simulink library "carnotUIBK_bus"  (R2023b)
settings: Solver=VariableStepAuto  StartTime=0.0  StopTime=10.0  RelTol=1e-3  EnableMultiTasking=on
values from neighbouring files (symbols this model uses):
  A = 7*10*2    (= 140)    [theta_ground_v1.m]    (also in xlswrite1.m = num2cell(data))
  amb_factor = 1    [DOOR.m]    (also in WALL.m; WINDOW.m = 0)
  area = obj.width * obj.height    [DOOR.m]    (also in RES.m = []; ROOM.m = 0; THERMALZONE.m = area + room(kk).area; WALL.m = area - obj.doors(jj).calc_area())
  B = A/(0.5 * P)    (= 8.23529411765)    [theta_ground_v1.m]
  boundary = BOUNDARY()    [BUILDING.m]    (also in WALL.m = '')
  building = obj    [BUILDING.m]    (also in create_building_automatic.m = building.save(); ini_building_automatic.m = building.add_variant_hvac(building.variant_hvac, hvac); load_building_automatic.m = building.save())
  C = zeros(1,length(d)+1)    [CONSTRUCTION.m]    (also in DOOR.m = [0 0 0]; WALL.m = [0 0 0]; WINDOW.m = [0 0 0])
  control = 2    [GAIN.m]    (also in GAINS.m)
  cp = str2num(value)    [CONSTRUCTION.m]
  height = 0    [DOOR.m]    (also in ROOM.m; THERMALZONE.m; WALL.m; WINDOW.m)
  p = [timevec_weather weather(:,12)]    [BOUNDARY.m]    (also in WEATHER.m = 0; init_carnotUIBK.m = cell2mat(carnotUIBKpaths(i,2)))
  rho = str2num(value)    [CONSTRUCTION.m]    (also in theta_ground_v1.m = 2000)
  type = 1    [CONSTRUCTION.m]    (also in GAINS.m = raw_moisture{ii,3}; STRUCTURE.m = 0)
  view_factor = 1    [DOOR.m]    (also in WINDOW.m = 0)
  wall = []    [ROOM.m]
  z = obj.Z    [WALL.m]    (also in theta_ground_v1.m = 0)
  zone = obj.zone(ind)    [THERMALZONE.m]
undefined symbols (not defined in the file or in its folder): const, Dd, get_building, mdot_air, mdot_CO2, mdot_H2O, mdot_VOC, pos, Qdot_C, Qdot_H, Qdot_I_electricity, Qdot_I_light, Qdot_I_person, Qdot_S, Qdot_T_ground, Qdot_T_internal, Qdot_T_neighbour, Qdot_T_opaque, Qdot_T_window, Qdot_V_infiltration, Qdot_V_mech, Qdot_V_window, Qdotc, Qdotr, r_frame, solar_ratio, solar_ratio1, solar_ratio2, Tc, Tr, Ts, Uvalue, wallsurface, window, window_height, window_heigth, window_width, windowsurface, x_CO2, x_H2O, x_VOC
libraries: $bdroot x134, carnot x87, simulink_extras x14, slpidlib x4, simulink x3
(part 4 of 12)

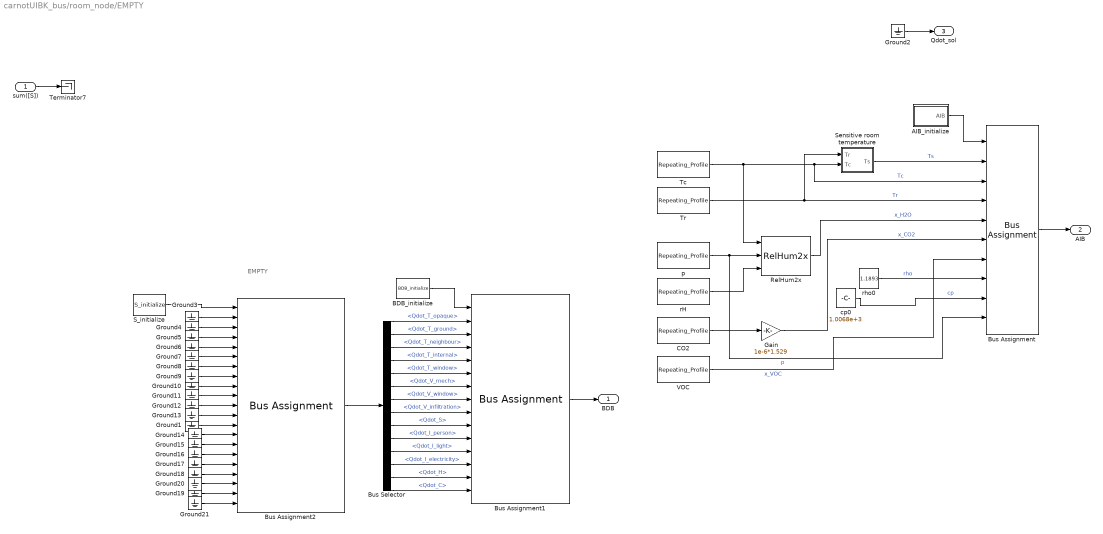
== system carnotUIBK_bus/room_node/EMPTY ==
  note: EMPTY
  sum([S]) : Inport
  AIB_initialize : Subsystem
  BDB_initialize : $bdroot/general/BDB_initialize  SystemSampleTime=-1  VariantActivationTime=update diagram  AllowFlexibleInterface=on  Latency=0  AutoFrameSizeCalculation=off
  Bus Assignment : BusAssignment  AssignedSignals=Ts,Tc,Tr,x_H2O,x_CO2,x_VOC,rho,cp,p
  Bus Assignment1 : BusAssignment  AssignedSignals=Qdot_T_opaque,Qdot_T_ground,Qdot_T_neighbour,Qdot_T_internal,Qdot_T_window,Qdot_V_mech,Qdot_V_window,Qdot_V_infiltration,Qdot_S,Qdot_I_person,Qdot_I_light,Qdot_I_electricity,Qdot_H,Qdot_C
  Bus Assignment2 : BusAssignment  AssignedSignals=Qdotc,Qdotr,Qdot_S,mdot_air,mdot_H2O,mdot_CO2,mdot_VOC,Qdot_T_opaque,Qdot_T_ground,Qdot_T_neighbour,Qdot_T_window,Qdot_T_internal,Qdot_V_mech,Qdot_V_window,Qdot_V_infiltration,Qdot_I_person,Qdot_I_light,Qdot_I_electricity,Qdot_H,Qdot_C
  Bus Selector : BusSelector  OutputSignals=Qdot_T_opaque,Qdot_T_ground,Qdot_T_neighbour,Qdot_T_internal,Qdot_T_window,Qdot_V_mech,Qdot_V_window,Qdot_V_infiltration,Qdot_S,Qdot_I_person,Qdot_I_light,Qdot_I_electricity,Qdot_H,Qdot_C
  CO2 : carnot/Load/General/Repeating_Profile  period=temperature_timevalues(end)  rep_seq_t=temperature_timevalues(1:end-1)  rep_seq_d=temperature_timeduration  rep_seq_y=temperature_CO2
      settings: SourceProductName=Carnot
  Gain : Gain  Gain=1e-6*1.529
  Ground{1..21} (21 alike) : Ground
  RelHum2x : carnot/Basic/Material_Properties/RelHum2x
      settings: SourceProductName=Carnot
  S_initialize : $bdroot/general/S_initialize  SystemSampleTime=-1  VariantActivationTime=update diagram  AllowFlexibleInterface=on  Latency=0  AutoFrameSizeCalculation=off
  Sensitive room temperature : Subsystem  mask(SENSITIVE TEMPERATURE){share_c=50}
      mask prompts: share_c "SHARE of convective part, [0,100%]:"
      mask help:
      | This block merges the convective and radiative zone node temperature to the SENSITIVE ZONE TEMPERATURE (weighted arithmetic average of both components).
      |
      | [T] = [Tc; Tr]:  temperature vector of node, °C
      | Ts:              sensitive zone temperature, °C
      mask init: same as carnotUIBK_bus/room_node/2-node/Sensitive room temperature
  Tc : carnot/Load/General/Repeating_Profile  period=temperature_timevalues(end)  rep_seq_t=temperature_timevalues(1:end-1)  rep_seq_d=temperature_timeduration  rep_seq_y=temperature_Tc
      settings: SourceProductName=Carnot
  Terminator7 : Terminator
  Tr : carnot/Load/General/Repeating_Profile  period=temperature_timevalues(end)  rep_seq_t=temperature_timevalues(1:end-1)  rep_seq_d=temperature_timeduration  rep_seq_y=temperature_Tr
      settings: SourceProductName=Carnot
  VOC : carnot/Load/General/Repeating_Profile  period=temperature_timevalues(end)  rep_seq_t=temperature_timevalues(1:end-1)  rep_seq_d=temperature_timeduration  rep_seq_y=temperature_VOC
      settings: SourceProductName=Carnot
  cp0 : Constant  Value=1.0068e+3
  p : carnot/Load/General/Repeating_Profile  period=temperature_timevalues(end)  rep_seq_t=temperature_timevalues(1:end-1)  rep_seq_d=temperature_timeduration  rep_seq_y=temperature_p
      settings: SourceProductName=Carnot
  rH : carnot/Load/General/Repeating_Profile  period=temperature_timevalues(end)  rep_seq_t=temperature_timevalues(1:end-1)  rep_seq_d=temperature_timeduration  rep_seq_y=temperature_rH
      settings: SourceProductName=Carnot
  rho0 : Constant  Value=1.1893
  BDB : Outport  VectorParamsAs1DForOutWhenUnconnected=off
  AIB : Outport  Port=2  VectorParamsAs1DForOutWhenUnconnected=off
  Qdot_sol : Outport  Port=3  VectorParamsAs1DForOutWhenUnconnected=off
  wires:
  Ground2/1 -> Qdot_sol/1
  cp0/1 -> Bus Assignment/9  "cp"
  rho0/1 -> Bus Assignment/8  "rho"
  p/1 -> Bus Assignment/10, RelHum2x/2  "p"
  VOC/1 -> Bus Assignment/7  "x_VOC"
  Tc/1 -> RelHum2x/1, Bus Assignment/3, Sensitive room temperature/2(Tc)  "Tc"
  Tr/1 -> Bus Assignment/4, Sensitive room temperature/1(Tr)  "Tr"
  RelHum2x/1 -> Bus Assignment/5  "x_H2O"
  Gain/1 -> Bus Assignment/6  "x_CO2"
  Sensitive room temperature/1(Ts) -> Bus Assignment/2  "Ts"
  rH/1 -> RelHum2x/3
  CO2/1 -> Gain/1
  Bus Assignment/1 -> AIB/1
  AIB_initialize/1(AIB) -> Bus Assignment/1
  BDB_initialize/1 -> Bus Assignment1/1
  Bus Assignment1/1 -> BDB/1
  sum([S])/1 -> Terminator7/1
  S_initialize/1 -> Bus Assignment2/1
  Ground3/1 -> Bus Assignment2/2
  Ground4/1 -> Bus Assignment2/3
  Ground5/1 -> Bus Assignment2/4
  Ground6/1 -> Bus Assignment2/5
  Ground7/1 -> Bus Assignment2/6
  Ground8/1 -> Bus Assignment2/7
  Ground9/1 -> Bus Assignment2/8
  Ground10/1 -> Bus Assignment2/9
  Ground11/1 -> Bus Assignment2/10
  Ground12/1 -> Bus Assignment2/11
  Ground13/1 -> Bus Assignment2/12
  Ground14/1 -> Bus Assignment2/14
  Ground15/1 -> Bus Assignment2/15
  Ground16/1 -> Bus Assignment2/16
  Ground17/1 -> Bus Assignment2/17
  Ground18/1 -> Bus Assignment2/18
  Ground20/1 -> Bus Assignment2/19
  Ground19/1 -> Bus Assignment2/20
  Ground21/1 -> Bus Assignment2/21
  Bus Assignment2/1 -> Bus Selector/1
  Bus Selector/1 -> Bus Assignment1/2  "<Qdot_T_opaque>"
  Bus Selector/2 -> Bus Assignment1/3  "<Qdot_T_ground>"
  Bus Selector/3 -> Bus Assignment1/4  "<Qdot_T_neighbour>"
  Bus Selector/5 -> Bus Assignment1/6  "<Qdot_T_window>"
  Bus Selector/6 -> Bus Assignment1/7  "<Qdot_V_mech>"
  Bus Selector/7 -> Bus Assignment1/8  "<Qdot_V_window>"
  Bus Selector/8 -> Bus Assignment1/9  "<Qdot_V_infiltration>"
  Bus Selector/9 -> Bus Assignment1/10  "<Qdot_S>"
  Bus Selector/10 -> Bus Assignment1/11  "<Qdot_I_person>"
  Bus Selector/11 -> Bus Assignment1/12  "<Qdot_I_light>"
  Bus Selector/12 -> Bus Assignment1/13  "<Qdot_I_electricity>"
  Bus Selector/13 -> Bus Assignment1/14  "<Qdot_H>"
  Bus Selector/14 -> Bus Assignment1/15  "<Qdot_C>"
  Ground1/1 -> Bus Assignment2/13
  Bus Selector/4 -> Bus Assignment1/5  "<Qdot_T_internal>"

== system carnotUIBK_bus/wall_intersection/EMPTY ==
  AIB1 : Inport
  AIB2 : Inport  Port=2
  Qdot_sol1 : Inport  Port=3
  Qdot_sol2 : Inport  Port=4
  S_initialize : $bdroot/general/S_initialize  SystemSampleTime=-1  VariantActivationTime=update diagram  AllowFlexibleInterface=on  Latency=0  AutoFrameSizeCalculation=off
  S_initialize1 : $bdroot/general/S_initialize  SystemSampleTime=-1  VariantActivationTime=update diagram  AllowFlexibleInterface=on  Latency=0  AutoFrameSizeCalculation=off
  Terminator{,2,4..5} (4 alike) : Terminator
  solar_ratio1 : Gain  Gain=solar_ratio1
  solar_ratio2 : Gain  Gain=solar_ratio2
  "[S1]" : Outport  VectorParamsAs1DForOutWhenUnconnected=off
  "[S2]" : Outport  Port=2  VectorParamsAs1DForOutWhenUnconnected=off
  wires:
  solar_ratio1/1 -> Terminator4/1
  Qdot_sol1/1 -> solar_ratio1/1
  AIB1/1 -> Terminator2/1
  S_initialize/1 -> "[S1]"/1
  AIB2/1 -> Terminator/1
  solar_ratio2/1 -> Terminator5/1
  Qdot_sol2/1 -> solar_ratio2/1
  S_initialize1/1 -> "[S2]"/1

== system carnotUIBK_bus/wall_intersection/R-C model ==
  AIB1 : Inport
  AIB2 : Inport  Port=2
  Qdot_sol1 : Inport  Port=3
  Qdot_sol2 : Inport  Port=4
  Ground : Ground
  Terminator{,1..3,5} (5 alike) : Terminator
  Wall_basic1 : carnot/Basic/Thermal_Models/Wall_basic  tau=tau  t0=t0  d=d  dactive=dactive  cond=cond  cwall=cwall  rho=rho
      settings: SourceProductName=Carnot
  alpha_i1 : Subsystem  Variant=on  mask{view_factor=view_factor}
  alpha_i2 : Subsystem  Variant=on  mask{view_factor=amb_factor}
  nohygrothermal : Constant  Value=0
  solar_ratio1 : Gain  Gain=solar_ratio1
  solar_ratio2 : Gain  Gain=solar_ratio2
  "[S1]" : Outport  VectorParamsAs1DForOutWhenUnconnected=off
  "[S2]" : Outport  Port=2  VectorParamsAs1DForOutWhenUnconnected=off
  wires:
  alpha_i1/2("[S]") -> "[S1]"/1
  alpha_i1/3(alpha_c) -> Terminator/1
  nohygrothermal/1 -> alpha_i2/4(phis), alpha_i1/4(phis)
  solar_ratio1/1 -> alpha_i1/3(Qdot sol)
  Qdot_sol1/1 -> solar_ratio1/1
  alpha_i1/1(qdots) -> Wall_basic1/3
  alpha_i2/1(qdots) -> Wall_basic1/1
  Wall_basic1/3 -> alpha_i1/1(Ts)
  Wall_basic1/1 -> alpha_i2/1(Ts)
  Wall_basic1/2 -> Terminator5/1
  Ground/1 -> Wall_basic1/2
  Qdot_sol2/1 -> solar_ratio2/1
  AIB1/1 -> alpha_i1/2(AIB)
  AIB2/1 -> alpha_i2/2(AIB)
  solar_ratio2/1 -> alpha_i2/3(Qdot sol)
  alpha_i2/3(alpha_c) -> Terminator2/1
  alpha_i2/2("[S]") -> "[S2]"/1
  alpha_i1/4(phi_i_1/100) -> Terminator1/1
  alpha_i2/4(phi_i_1/100) -> Terminator3/1

== system carnotUIBK_bus/wall_intersection/UA ==
  AIB1 : Inport
  AIB2 : Inport  Port=2
  Qdot_sol1 : Inport  Port=3
  Qdot_sol2 : Inport  Port=4
  1/U : Constant  Value=1/U
  Add : Sum  Inputs=2
  Add1 : Sum  Inputs=+-
  Bus Assignment1 : BusAssignment  AssignedSignals=Qdotc,Qdotr,Qdot_T_neighbour
  Bus Assignment2 : BusAssignment  AssignedSignals=Qdotc,Qdotr,Qdot_T_neighbour
  Bus Selector1 : BusSelector  OutputSignals=Ts
  Bus Selector2 : BusSelector  OutputSignals=Ts
  Gain : Gain  Gain=-1
  Qdot : Sum  Inputs=2
  Qdot1 : Sum  Inputs=2
  Qdot_T : Product  Inputs=**/
  Qdotr/Qdotc : Gain  Gain=0.5
  Qdotr/Qdotc1 : Gain  Gain=0.5
  Rsi : Subsystem  Variant=on
  S_initialize : $bdroot/general/S_initialize  SystemSampleTime=-1  VariantActivationTime=update diagram  AllowFlexibleInterface=on  Latency=0  AutoFrameSizeCalculation=off
  S_initialize1 : $bdroot/general/S_initialize  SystemSampleTime=-1  VariantActivationTime=update diagram  AllowFlexibleInterface=on  Latency=0  AutoFrameSizeCalculation=off
  solar_ratio1 : Gain  Gain=solar_ratio1
  solar_ratio2 : Gain  Gain=solar_ratio2
  wallsurface : Constant  Value=wallsurface
  "[S1]" : Outport  VectorParamsAs1DForOutWhenUnconnected=off
  "[S2]" : Outport  Port=2  VectorParamsAs1DForOutWhenUnconnected=off
  wires:
  Qdot_sol1/1 -> solar_ratio1/1
  Qdot_sol2/1 -> solar_ratio2/1
  Bus Selector1/1 -> Add1/2  "<Ts>"
  Add1/1 -> Qdot_T/1
  Add/1 -> Qdot_T/3
  wallsurface/1 -> Qdot_T/2
  Rsi/1(Rsi) -> Add/2
  1/U/1 -> Add/1
  AIB1/1 -> Bus Selector1/1
  AIB2/1 -> Bus Selector2/1
  Bus Selector2/1 -> Add1/1  "<Ts>"
  Bus Assignment2/1 -> "[S1]"/1
  Qdotr/Qdotc/1 -> Bus Assignment2/2, Bus Assignment2/3
  solar_ratio1/1 -> Qdot/2
  Qdotr/Qdotc1/1 -> Bus Assignment1/3, Bus Assignment1/2
  Qdot1/1 -> Bus Assignment1/4, Qdotr/Qdotc1/1
  Gain/1 -> Qdot1/1
  solar_ratio2/1 -> Qdot1/2
  Qdot/1 -> Bus Assignment2/4, Qdotr/Qdotc/1
  Qdot_T/1 -> Gain/1, Qdot/1
  S_initialize/1 -> Bus Assignment2/1
  S_initialize1/1 -> Bus Assignment1/1
  Bus Assignment1/1 -> "[S2]"/1

== system carnotUIBK_bus/wall_intersection/hygrothermal model ==
  AIB1 : Inport
  AIB2 : Inport  Port=2
  Qdot_sol1 : Inport  Port=3
  Qdot_sol2 : Inport  Port=4
  Bus Selector : BusSelector  OutputSignals=Tc
  Bus Selector1 : BusSelector  OutputSignals=Tc
  Constant1 : Constant  Value=0
  Constant2 : Constant  Value=0
  S-Function1 : S-Function  FunctionName=pdepesim_hygro_c_v4  Parameters=xmesh,length(xmesh),X(2:end),length(d),lambda,rho,cp,mu,ufs,FSF_u,FSF_phi,FSF_dudphi,FSF_k,K_kleff,K_u,K_kl,FSF_length,K_length,T_ini,Phi_ini,T_source,Phi_source,Tdactive,Phidactive  SFunctionDeploymentMode=off  EnableBusSupport=off
  Terminator{1..6} (6 alike) : Terminator
  alpha_i1 : Subsystem  Variant=on  mask{view_factor=view_factor}
  alpha_i2 : Subsystem  Variant=on  mask{view_factor=amb_factor}
  solar_ratio1 : Gain  Gain=solar_ratio1
  solar_ratio2 : Gain  Gain=solar_ratio2
  "[S1]" : Outport  VectorParamsAs1DForOutWhenUnconnected=off
  "[S2]" : Outport  Port=2  VectorParamsAs1DForOutWhenUnconnected=off
  wires:
  S-Function1/6 -> alpha_i1/4(phis)
  S-Function1/5 -> alpha_i2/4(phis)
  S-Function1/4 -> alpha_i1/1(Ts)
  S-Function1/3 -> alpha_i2/1(Ts)
  S-Function1/8 -> Terminator3/1
  S-Function1/7 -> Terminator4/1
  S-Function1/2 -> Terminator5/1
  S-Function1/1 -> Terminator6/1
  S-Function1/9 -> Terminator2/1
  S-Function1/10 -> Terminator1/1
  Constant1/1 -> S-Function1/10
  Constant2/1 -> S-Function1/9
  alpha_i1/3(alpha_c) -> S-Function1/8
  alpha_i2/3(alpha_c) -> S-Function1/7
  alpha_i1/4(phi_i_1/100) -> S-Function1/6
  Bus Selector/1 -> S-Function1/5  "<Tc>"
  alpha_i2/4(phi_i_1/100) -> S-Function1/4
  Bus Selector1/1 -> S-Function1/3  "<Tc>"
  alpha_i1/1(qdots) -> S-Function1/2
  alpha_i2/1(qdots) -> S-Function1/1
  solar_ratio1/1 -> alpha_i1/3(Qdot sol)
  Qdot_sol1/1 -> solar_ratio1/1
  AIB1/1 -> alpha_i1/2(AIB), Bus Selector/1
  alpha_i1/2("[S]") -> "[S1]"/1
  Qdot_sol2/1 -> solar_ratio2/1
  solar_ratio2/1 -> alpha_i2/3(Qdot sol)
  AIB2/1 -> Bus Selector1/1, alpha_i2/2(AIB)
  alpha_i2/2("[S]") -> "[S2]"/1

== system carnotUIBK_bus/wall_zone/EMPTY ==
  WDB : Inport
  GDB : Inport  Port=2
  NDB : Inport  Port=3
  AIB : Inport  Port=4
  Qdot_in : Inport  Port=5
  Qdot_sol : Inport  Port=6
  Bus Assignment2 : BusAssignment  AssignedSignals=Qdotc,Qdotr,Qdot_S,mdot_air,mdot_H2O,mdot_CO2,mdot_VOC,Qdot_T_opaque,Qdot_T_ground,Qdot_T_neighbour,Qdot_T_window,Qdot_V_mech,Qdot_V_window,Qdot_V_infiltration,Qdot_I_person,Qdot_I_light,Qdot_I_electricity,Qdot_H,Qdot_C
  Constant{1..19} (19 alike) : Constant  Value=0
  Ground3 : Ground
  S_initialize : $bdroot/general/S_initialize  SystemSampleTime=-1  VariantActivationTime=update diagram  AllowFlexibleInterface=on  Latency=0  AutoFrameSizeCalculation=off
  Terminator{,1..5} (6 alike) : Terminator
  solar_ratio : Gain  Gain=solar_ratio
  "[S]" : Outport  VectorParamsAs1DForOutWhenUnconnected=off
  theta_out : Outport  Port=2  VectorParamsAs1DForOutWhenUnconnected=off
  wires:
  NDB/1 -> Terminator1/1
  GDB/1 -> Terminator/1
  Bus Assignment2/1 -> "[S]"/1
  Ground3/1 -> theta_out/1
  WDB/1 -> Terminator2/1
  AIB/1 -> Terminator3/1
  Qdot_sol/1 -> solar_ratio/1
  Qdot_in/1 -> Terminator5/1
  solar_ratio/1 -> Terminator4/1
  S_initialize/1 -> Bus Assignment2/1
  Constant3/1 -> Bus Assignment2/2
  Constant1/1 -> Bus Assignment2/3
  Constant4/1 -> Bus Assignment2/4
  Constant2/1 -> Bus Assignment2/5
  Constant7/1 -> Bus Assignment2/6
  Constant5/1 -> Bus Assignment2/7
  Constant8/1 -> Bus Assignment2/8
  Constant6/1 -> Bus Assignment2/9
  Constant11/1 -> Bus Assignment2/10
  Constant9/1 -> Bus Assignment2/11
  Constant12/1 -> Bus Assignment2/12
  Constant10/1 -> Bus Assignment2/13
  Constant15/1 -> Bus Assignment2/14
  Constant13/1 -> Bus Assignment2/15
  Constant16/1 -> Bus Assignment2/16
  Constant14/1 -> Bus Assignment2/17
  Constant17/1 -> Bus Assignment2/18
  Constant19/1 -> Bus Assignment2/19
  Constant18/1 -> Bus Assignment2/20

== system carnotUIBK_bus/wall_zone/R-C model ==
  WDB : Inport
  GDB : Inport  Port=2
  NDB : Inport  Port=3
  AIB : Inport  Port=4
  Qdot_in : Inport  Port=5
  Qdot_sol : Inport  Port=6
  Bus Assignment2 : BusAssignment  AssignedSignals=Qdot_H
  Bus to Vector : BusToVector
  Bus to Vector1 : BusToVector
  S_initialize : $bdroot/general/S_initialize  SystemSampleTime=-1  VariantActivationTime=update diagram  AllowFlexibleInterface=on  Latency=0  AutoFrameSizeCalculation=off
  Selector1 : Selector  InputPortWidth=6  IndexOptions=Index vector (dialog)  Indices=[boundary]  OutputSizes=1
  Selector2 : Selector  InputPortWidth=6  IndexOptions=Index vector (dialog)  Indices=[boundary]  OutputSizes=1
  Selector4 : Selector  InputPortWidth=NUMBEROFWINDOWSINZONESANDINTERSECTIONS  IndexOptions=Index vector (dialog)  Indices=[wall]  OutputSizes=1
  Ssum : $bdroot/general/Ssum  SystemSampleTime=-1  VariantActivationTime=update diagram  AllowFlexibleInterface=on  Latency=0  AutoFrameSizeCalculation=off
  Terminator{,1..4} (5 alike) : Terminator
  Wall_basic : carnot/Basic/Thermal_Models/Wall_basic  tau=tau  t0=t0  d=d  dactive=dactive  cond=cond  cwall=cwall  rho=rho
      settings: SourceProductName=Carnot
  alpha_e : Subsystem  Variant=on
  alpha_i : Subsystem  Variant=on  mask{view_factor=view_factor}
  nohygrothermal : Constant  Value=0
  per surface : Gain  Gain=1/wallsurface  SaturateOnIntegerOverflow=on  OutDataTypeStr=Inherit: Same as input  ParamDataTypeStr=Inherit: Same as input
  solar_ratio : Gain  Gain=solar_ratio
  "[S]" : Outport  VectorParamsAs1DForOutWhenUnconnected=off
  theta_out : Outport  Port=2  VectorParamsAs1DForOutWhenUnconnected=off
  wires:
  per surface/1 -> Wall_basic/2
  Wall_basic/2 -> theta_out/1
  WDB/1 -> alpha_e/1(WDB)
  Qdot_in/1 -> Selector4/1
  Wall_basic/1 -> alpha_e/5(Ts)
  Wall_basic/3 -> alpha_i/1(Ts)
  AIB/1 -> alpha_i/2(AIB), alpha_e/4(AIB)
  alpha_e/1(qdots) -> Wall_basic/1
  alpha_i/1(qdots) -> Wall_basic/3
  Qdot_sol/1 -> solar_ratio/1
  Selector4/1 -> Bus Assignment2/2, per surface/1
  Bus to Vector/1 -> Selector1/1
  Bus to Vector1/1 -> Selector2/1
  GDB/1 -> Bus to Vector/1
  NDB/1 -> Bus to Vector1/1
  solar_ratio/1 -> alpha_i/3(Qdot sol), alpha_e/6(Qdot_sol)
  nohygrothermal/1 -> alpha_i/4(phis), alpha_e/7(phis)
  alpha_i/3(alpha_c) -> Terminator/1
  alpha_i/4(phi_i_1/100) -> Terminator1/1
  alpha_i/2("[S]") -> Ssum/2
  Ssum/1 -> "[S]"/1
  Selector1/1 -> alpha_e/2(GDB)
  Selector2/1 -> alpha_e/3(NDB)
  alpha_e/2("[S]") -> Ssum/1
  alpha_e/3(alpha_c) -> Terminator2/1
  alpha_e/4(phi_e_1/100) -> Terminator3/1
  Bus Assignment2/1 -> Ssum/3
  alpha_e/5(theta_e) -> Terminator4/1
  S_initialize/1 -> Bus Assignment2/1

== system carnotUIBK_bus/wall_zone/UA ==
  WDB : Inport
  GDB : Inport  Port=2
  NDB : Inport  Port=3
  AIB : Inport  Port=4
  Qdot_in : Inport  Port=5
  Qdot_sol : Inport  Port=6
  1/U : Constant  Value=1/U
  Bus to Vector : BusToVector
  Bus to Vector1 : BusToVector
  Ground : Ground
  Rse : Subsystem  Variant=on
  Rsi : Subsystem  Variant=on
  Selector : Selector  InputPortWidth=6  IndexOptions=Index vector (dialog)  Indices=[boundary]  OutputSizes=1
  Selector1 : Selector  InputPortWidth=6  IndexOptions=Index vector (dialog)  Indices=[boundary]  OutputSizes=1
  Selector2 : Selector  InputPortWidth=NUMBEROFWINDOWSINZONESANDINTERSECTIONS  IndexOptions=Index vector (dialog)  Indices=[wall]  OutputSizes=1
  solar_ratio : Gain  Gain=solar_ratio
  "[S]" : Outport  VectorParamsAs1DForOutWhenUnconnected=off
  theta_out : Outport  Port=2  VectorParamsAs1DForOutWhenUnconnected=off
  wires:
  NDB/1 -> Bus to Vector1/1
  GDB/1 -> Bus to Vector/1
  WDB/1 -> Rse/1(WDB)
  Rse/1("[S]") -> "[S]"/1
  Ground/1 -> theta_out/1
  AIB/1 -> Rse/4(AIB)
  Qdot_sol/1 -> solar_ratio/1
  1/U/1 -> Rse/7(R)
  Rsi/1(Rsi) -> Rse/8(Rsi)
  Qdot_in/1 -> Selector2/1
  Bus to Vector/1 -> Selector/1
  Bus to Vector1/1 -> Selector1/1
  Selector/1 -> Rse/2(GDB)
  Selector1/1 -> Rse/3(NDB)
  Selector2/1 -> Rse/6(Qdot_in)
  solar_ratio/1 -> Rse/5(Qdot_sol)

== system carnotUIBK_bus/wall_zone/hygrothermal model ==
  WDB : Inport
  GDB : Inport  Port=2
  NDB : Inport  Port=3
  AIB : Inport  Port=4
  Qdot_in : Inport  Port=5
  Qdot_sol : Inport  Port=6
  Bus Assignment2 : BusAssignment  AssignedSignals=Qdot_H
  Bus Selector : BusSelector  OutputSignals=Tc
  Bus to Vector : BusToVector
  Bus to Vector1 : BusToVector
  Constant1 : Constant  Value=0
  Constant2 : Constant  Value=0
  S-Function1 : S-Function  FunctionName=pdepesim_hygro_c_v4  Parameters=xmesh,length(xmesh),X(2:end),length(d),lambda,rho,cp,mu,ufs,FSF_u,FSF_phi,FSF_dudphi,FSF_k,K_kleff,K_u,K_kl,FSF_length,K_length,T_ini,Phi_ini,T_source,Phi_source,Tdactive,Phidactive  SFunctionDeploymentMode=off  EnableBusSupport=off
  S_initialize : $bdroot/general/S_initialize  SystemSampleTime=-1  VariantActivationTime=update diagram  AllowFlexibleInterface=on  Latency=0  AutoFrameSizeCalculation=off
  Selector1 : Selector  InputPortWidth=6  IndexOptions=Index vector (dialog)  Indices=[boundary]  OutputSizes=1
  Selector2 : Selector  InputPortWidth=6  IndexOptions=Index vector (dialog)  Indices=[boundary]  OutputSizes=1
  Selector4 : Selector  InputPortWidth=NUMBEROFWINDOWSINZONESANDINTERSECTIONS  IndexOptions=Index vector (dialog)  Indices=[wall]  OutputSizes=1
  Ssum : $bdroot/general/Ssum  SystemSampleTime=-1  VariantActivationTime=update diagram  AllowFlexibleInterface=on  Latency=0  AutoFrameSizeCalculation=off
  Terminator{,1..6} (7 alike) : Terminator
  alpha_e : Subsystem  Variant=on
  alpha_i : Subsystem  Variant=on  mask{view_factor=view_factor}
  per surface : Gain  Gain=1/wallsurface  SaturateOnIntegerOverflow=on  OutDataTypeStr=Inherit: Same as input  ParamDataTypeStr=Inherit: Same as input
  solar_ratio : Gain  Gain=solar_ratio
  "[S]" : Outport  VectorParamsAs1DForOutWhenUnconnected=off
  theta_out : Outport  Port=2  VectorParamsAs1DForOutWhenUnconnected=off
  wires:
  WDB/1 -> alpha_e/1(WDB)
  Qdot_in/1 -> Selector4/1
  AIB/1 -> alpha_e/4(AIB), Bus Selector/1, alpha_i/2(AIB)
  Qdot_sol/1 -> solar_ratio/1
  Selector4/1 -> Bus Assignment2/2, per surface/1
  Bus to Vector/1 -> Selector1/1
  Bus to Vector1/1 -> Selector2/1
  GDB/1 -> Bus to Vector/1
  NDB/1 -> Bus to Vector1/1
  solar_ratio/1 -> alpha_e/6(Qdot_sol), alpha_i/3(Qdot sol)
  alpha_i/2("[S]") -> Ssum/2
  Ssum/1 -> "[S]"/1
  Selector1/1 -> alpha_e/2(GDB)
  Selector2/1 -> alpha_e/3(NDB)
  alpha_e/2("[S]") -> Ssum/1
  Bus Assignment2/1 -> Ssum/3
  alpha_e/1(qdots) -> S-Function1/1
  alpha_i/1(qdots) -> S-Function1/2
  alpha_e/5(theta_e) -> S-Function1/3
  alpha_e/4(phi_e_1/100) -> S-Function1/4
  Bus Selector/1 -> S-Function1/5  "<Tc>"
  alpha_i/4(phi_i_1/100) -> S-Function1/6
  alpha_e/3(alpha_c) -> S-Function1/7
  alpha_i/3(alpha_c) -> S-Function1/8
  per surface/1 -> Terminator/1
  Constant2/1 -> S-Function1/9
  Constant1/1 -> S-Function1/10
  S-Function1/10 -> Terminator1/1
  S-Function1/9 -> Terminator2/1
  S-Function1/1 -> Terminator6/1
  S-Function1/2 -> Terminator5/1
  S-Function1/7 -> Terminator4/1
  S-Function1/8 -> Terminator3/1
  S-Function1/3 -> alpha_e/5(Ts)
  S-Function1/4 -> alpha_i/1(Ts)
  S-Function1/5 -> alpha_e/7(phis)
  S-Function1/6 -> alpha_i/4(phis)
  S_initialize/1 -> Bus Assignment2/1

== system carnotUIBK_bus/window/EMTPY ==
  WDB : Inport
  AIB : Inport  Port=2
  control : Inport  Port=3
  S_initialize : $bdroot/general/S_initialize  SystemSampleTime=-1  VariantActivationTime=update diagram  AllowFlexibleInterface=on  Latency=0  AutoFrameSizeCalculation=off
  Selector1 : Selector  InputPortWidth=NUMBEROFCONTROLS  IndexOptions=Index vector (dialog)  Indices=[control]  OutputSizes=1
  Terminator1 : Terminator
  Terminator2 : Terminator
  Terminator4 : Terminator
  "[S]" : Outport  VectorParamsAs1DForOutWhenUnconnected=off
  wires:
  S_initialize/1 -> "[S]"/1
  control/1 -> Selector1/1
  AIB/1 -> Terminator1/1
  WDB/1 -> Terminator2/1
  Selector1/1 -> Terminator4/1

== system carnotUIBK_bus/window/window_CARNOT ==
  WDB : Inport
  AIB : Inport  Port=2
  control : Inport  Port=3
  Add : Sum  Inputs=+-
  Constant : Constant
  Product : Product
  S_initialize1 : $bdroot/general/S_initialize  SystemSampleTime=-1  VariantActivationTime=update diagram  AllowFlexibleInterface=on  Latency=0  AutoFrameSizeCalculation=off
  Selector1 : Selector  InputPortWidth=NUMBEROFCONTROLS  IndexOptions=Index vector (dialog)  Indices=[control]  OutputSizes=1
  Ssum : $bdroot/general/Ssum  SystemSampleTime=-1  VariantActivationTime=update diagram  AllowFlexibleInterface=on  Latency=0  AutoFrameSizeCalculation=off
  Terminator1 : Terminator
  Wall_basic : carnot/Basic/Thermal_Models/Wall_basic  tau=3600  t0=20  d=[0.1 0.1 0.1]  dactive=-1  cond=[1 2 1]  cwall=[800 1000 800]  rho=[2000 2700 2000]
      settings: SourceProductName=Carnot
  alfa_window_in : Subsystem  mask(ALFA){}
      mask help:
      | Convective and radiative heat transfer at the INDOOR SURFACE OF A VERTICAL WINDOW with 1-4 layers (each 3 ... 8 mm thick).
      |
      | Ts  : temperature of window surface, °C,
      | [sun_t]  : sun data (incidence angle, direct and diffuse radiation
      |     at tilted window surface),
      | [AIV]  : conditions of zone node,
      | qdots  : specific heat flow into window construction, W/m^2,
      | qdot_abs : specific irradiation absorption within window
      |     construction,  W/m^2,
      | [S]  : heat and air flow to zone node.
  alfa_window_out : Subsystem  mask(ALFA){}
      mask help:
      | Convective and radiative heat transfer at the OUTDOOR SURFACE OF A VERTICAL WINDOW.
      |
      | [W*] : modified weather data, adapted to height over ground,
      | Ts : temperature of outdoor window surface, °C,
      | qdots : specific heat flow into window construction, W/m^2,
      | [sun_t] : sun data (incidence angle, direct and diffuse radiation
      |                  at tilted window surface).
  position1 : Constant
  "[S]" : Outport  VectorParamsAs1DForOutWhenUnconnected=off
  wires:
  Wall_basic/1 -> alfa_window_out/3(Ts1)
  AIB/1 -> alfa_window_in/3("[AIV]")
  alfa_window_in/1(qdots2) -> Wall_basic/3
  WDB/1 -> alfa_window_out/1(WDB)
  alfa_window_out/1("[sun_t]") -> alfa_window_in/2("[sun_t]")
  Wall_basic/2 -> Terminator1/1
  alfa_window_out/2(qdots1) -> Wall_basic/1
  Wall_basic/3 -> alfa_window_in/1(Ts2)
  alfa_window_in/2(qdot_abs) -> Wall_basic/2
  position1/1 -> Product/1
  Product/1 -> alfa_window_out/2(g)
  control/1 -> Selector1/1
  Add/1 -> Product/2
  Constant/1 -> Add/1
  alfa_window_in/3("[S]") -> Ssum/2
  Ssum/1 -> "[S]"/1
  alfa_window_out/3("[S]") -> Ssum/1
  Selector1/1 -> Add/2
  S_initialize1/1 -> Ssum/3

== system carnotUIBK_bus/window/window_TF ==
  WDB : Inport
  AIB : Inport  Port=2
  control : Inport  Port=3
  Add : Sum  Inputs=+-
  Constant : Constant
  Constant1 : Constant  Value=0
  Product : Product  Inputs=4
  S_initialize1 : $bdroot/general/S_initialize  SystemSampleTime=-1  VariantActivationTime=update diagram  AllowFlexibleInterface=on  Latency=0  AutoFrameSizeCalculation=off
  Selector1 : Selector  InputPortWidth=NUMBEROFCONTROLS  IndexOptions=Index vector (dialog)  Indices=[control]  OutputSizes=1
  Ssum : $bdroot/general/Ssum  SystemSampleTime=-1  VariantActivationTime=update diagram  AllowFlexibleInterface=on  Latency=0  AutoFrameSizeCalculation=off
  alfa_window_in : Subsystem  mask(ALFA){}
      mask help:
      | Convective and radiative heat transfer at the INDOOR SURFACE OF A VERTICAL WINDOW with 1-4 layers (each 3 ... 8 mm thick).
      |
      | Ts  : temperature of window surface, °C,
      | [sun_t]  : sun data (incidence angle, direct and diffuse radiation
      |     at tilted window surface),
      | [AIV]  : conditions of zone node,
      | qdots  : specific heat flow into window construction, W/m^2,
      | [S]  : heat and air flow to zone node.
  alfa_window_out : Subsystem  mask(ALFA){}
      mask help:
      | Convective and radiative heat transfer at the OUTDOOR SURFACE OF A VERTICAL WINDOW.
      |
      | [W*] : modified weather data, adapted to height over ground,
      | Ts : temperature of outdoor window surface, °C,
      | qdots : specific heat flow into window construction, W/m^2,
      | [sun_t] : sun data (incidence angle, direct and diffuse radiation
      |                  at tilted window surface).
  lambda_window : Subsystem  mask(LAMBDA){}
      mask help:
      | Heat conduction through a transparent component (window).
      |
      | qdots1	: specific heat flow vertical on surface 1, W/m²
      | qdots2	: specific heat flow vertical on surface 2, W/m²
      | Ts1	: temperature of surface 1, °C
      | Ts2	: temperature of surface 2, °C
      |
      | NOTE CONVENTION for INPUT NUMBER:
      | "1"	  indoor surface of an outer window OR
      | 	  surface "a" of an inner window OR
      |  	  surface "f" of a glass floor
      |
      | "2"	  outdoor surface of a window OR
      | 	  surface "b" of an inner window OR
      |  	  surface "c" of a glass ceiling
  position1 : Constant  Value=zone{window,15}
  position2 : Constant
  time_value : FromWorkspace  VariableName=z.win_factor_seq{window}
  "[S]" : Outport  VectorParamsAs1DForOutWhenUnconnected=off
  wires:
  alfa_window_out/1("[sun_t]") -> alfa_window_in/2("[sun_t]")
  alfa_window_out/2(qdots1) -> lambda_window/1(qdots1)
  alfa_window_in/1(qdots2) -> lambda_window/2(qdots2)
  AIB/1 -> alfa_window_in/3("[AIV]")
  WDB/1 -> alfa_window_out/1(WDB), alfa_window_in/4(WDB)
  Ssum/1 -> "[S]"/1
  alfa_window_in/2("[S]") -> Ssum/2
  alfa_window_out/3("[S]") -> Ssum/1
  lambda_window/1(Ts1) -> alfa_window_out/3(Ts1)
  lambda_window/2(Ts2) -> alfa_window_in/1(Ts2)
  position2/1 -> Product/3
  control/1 -> Selector1/1
  Add/1 -> Product/4
  Constant/1 -> Add/1
  Product/1 -> alfa_window_out/2(g)
  Constant1/1 -> alfa_window_in/5(control)
  Selector1/1 -> Add/2
  time_value/1 -> Product/2
  position1/1 -> Product/1
  S_initialize1/1 -> Ssum/3

== system carnotUIBK_bus/window/window_TF_shading ==
  WDB : Inport
  AIB : Inport  Port=2
  control : Inport  Port=3
  Product : Product  Inputs=3
  S_initialize1 : $bdroot/general/S_initialize  SystemSampleTime=-1  VariantActivationTime=update diagram  AllowFlexibleInterface=on  Latency=0  AutoFrameSizeCalculation=off
  Selector1 : Selector  InputPortWidth=NUMBEROFCONTROLS  IndexOptions=Index vector (dialog)  Indices=[control]  OutputSizes=1
  Ssum : $bdroot/general/Ssum  SystemSampleTime=-1  VariantActivationTime=update diagram  AllowFlexibleInterface=on  Latency=0  AutoFrameSizeCalculation=off
  alfa_window_in : Subsystem  mask(ALFA){}
      mask help:
      | Convective and radiative heat transfer at the INDOOR SURFACE OF A VERTICAL WINDOW with 1-4 layers (each 3 ... 8 mm thick).
      |
      | Ts  : temperature of window surface, °C,
      | [sun_t]  : sun data (incidence angle, direct and diffuse radiation
      |     at tilted window surface),
      | [AIV]  : conditions of zone node,
      | qdots  : specific heat flow into window construction, W/m^2,
      | [S]  : heat and air flow to zone node.
  alfa_window_out : Subsystem  mask(ALFA){}
      mask help:
      | Convective and radiative heat transfer at the OUTDOOR SURFACE OF A VERTICAL WINDOW.
      |
      | [W*] : modified weather data, adapted to height over ground,
      | Ts : temperature of outdoor window surface, °C,
      | qdots : specific heat flow into window construction, W/m^2,
      | [sun_t] : sun data (incidence angle, direct and diffuse radiation
      |                  at tilted window surface).
  lambda_window : Subsystem  mask(LAMBDA){}
      mask help:
      | Heat conduction through a transparent component (window).
      |
      | qdots1	: specific heat flow vertical on surface 1, W/m²
      | qdots2	: specific heat flow vertical on surface 2, W/m²
      | Ts1	: temperature of surface 1, °C
      | Ts2	: temperature of surface 2, °C
      |
      | NOTE CONVENTION for INPUT NUMBER:
      | "1"	  indoor surface of an outer window OR
      | 	  surface "a" of an inner window OR
      |  	  surface "f" of a glass floor
      |
      | "2"	  outdoor surface of a window OR
      | 	  surface "b" of an inner window OR
      |  	  surface "c" of a glass ceiling
  position1 : Constant
  position2 : Constant  Value=zone{window,15}
  time_value : FromWorkspace  VariableName=z.win_factor_seq{window}
  "[S]" : Outport  VectorParamsAs1DForOutWhenUnconnected=off
  wires:
  position1/1 -> Product/3
  control/1 -> Selector1/1
  alfa_window_out/1("[sun_t]") -> alfa_window_in/2("[sun_t]")
  alfa_window_out/2(qdots1) -> lambda_window/1(qdots1)
  alfa_window_in/1(qdots2) -> lambda_window/2(qdots2)
  AIB/1 -> alfa_window_in/3("[AIV]")
  WDB/1 -> alfa_window_in/4(WDB), alfa_window_out/1(WDB)
  Ssum/1 -> "[S]"/1
  alfa_window_in/2("[S]") -> Ssum/2
  alfa_window_out/3("[S]") -> Ssum/1
  lambda_window/1(Ts1) -> alfa_window_out/3(Ts1)
  lambda_window/2(Ts2) -> alfa_window_in/1(Ts2)
  Selector1/1 -> alfa_window_in/5(control)
  time_value/1 -> Product/2
  position2/1 -> Product/1
  Product/1 -> alfa_window_out/2(g)
  S_initialize1/1 -> Ssum/3

== system carnotUIBK_bus/HVAC/HVAC_1001_electrical heaters/electrical heater zone 1 ==
  temperature setpoint : Inport
  temperature room : Inport  Port=2
  Enable : EnablePort
  Bus Assignment2 : BusAssignment  AssignedSignals=Qdotc,Qdotr,Qdot_H
  Bus Creator1 : BusCreator  Inputs=2
  Bus Selector5 : BusSelector  OutputSignals=Ts
  Integrator : Integrator
  PID : slpidlib/PID Controller  Controller=PI  Form=Ideal  TimeDomain=Continuous-time  UseExternalTs=off  SampleTime=-1  IntegratorMethod=Forward Euler  FilterMethod=Forward Euler  ControllerParametersSource=internal  P=Kp  I=1/(Tn*60)  UseKiTs=off  D=0  N=100  UseFilter=on  TunerSelectOption=Transfer Function Based (PID Tuner App)  InitialConditionSource=internal  InitialConditionForIntegrator=0  InitialConditionForFilter=0  DifferentiatorICPrevScaledInput=0  ExternalReset=none  TrackingMode=off  Kt=1  LimitOutput=on  SatLimitsSource=internal  UpperSaturationLimit=1  LowerSaturationLimit=0  LinearizeAsGain=off  AntiWindupMode=clamping  Kb=1  LimitIntegrator=off  UpperIntegratorSaturationLimit=inf  LowerIntegratorSaturationLimit=-inf  POutMin=[]  POutMax=[]  IOutMin=[]  IOutMax=[]  DOutMin=[]  DOutMax=[]  NOutMin=[]  NOutMax=[]  SumOutMin=[]  SumOutMax=[]  SaturationOutMin=[]  SaturationOutMax=[]  PParamMin=[]  PParamMax=[]  IParamMin=[]  IParamMax=[]  DParamMin=[]  DParamMax=[]  NParamMin=[]  NParamMax=[]  KbParamMin=[]  KbParamMax=[]  KtParamMin=[]  KtParamMax=[]  KbOutMin=[]  KbOutMax=[]  KtOutMin=[]  KtOutMax=[]  IntegratorOutMin=[]  IntegratorOutMax=[]  FilterOutMin=[]  FilterOutMax=[]  SumI1OutMin=[]  SumI1OutMax=[]  SumI2OutMin=[]  SumI2OutMax=[]  SumI3OutMin=[]  SumI3OutMax=[]  SumI4OutMin=[]  SumI4OutMax=[]  SumDOutMin=[]  SumDOutMax=[]  DifferentiatorOutMin=[]  DifferentiatorOutMax=[]  FilterDiffOutCoefMin=[]  FilterDiffOutCoefMax=[]  ReciprocalOutMin=[]  ReciprocalOutMax=[]  SumDenOutMin=[]  SumDenOutMax=[]  SumNumOutMin=[]  SumNumOutMax=[]  DivideOutMin=[]  DivideOutMax=[]  UdiffTsProdOutMin=[]  UdiffTsProdOutMax=[]  NTsProdOutMin=[]  NTsProdOutMax=[]  UintegralTsProdOutMin=[]  UintegralTsProdOutMax=[]  UngainTsProdOutMin=[]  UngainTsProdOutMax=[]  ClampingZeroOutDataTypeStr=Inherit: Inherit via back propagation  ClampingZeroOutMin=[]  ClampingZeroOutMax=[]  FilterDenConstantOutDataTypeStr=Inherit: Inherit via back propagation  FilterDenConstantOutMin=[]  FilterDenConstantOutMax=[]  PCopyOutDataTypeStr=Inherit: Inherit via back propagation  PCopyOutMin=[]  PCopyOutMax=[]  NCopyOutDataTypeStr=Inherit: Inherit via back propagation  NCopyOutMin=[]  NCopyOutMax=[]  IntegratorContinuousStateAttributes=''  IntegratorStateMustResolveToSignalObject=off  IntegratorRTWStateStorageClass=Auto  FilterContinuousStateAttributes=''  FilterStateMustResolveToSignalObject=off  FilterRTWStateStorageClass=Auto  ParallelPVariant=Passthrough  IdealPVariant=InternalParameters  IVariant=InternalParameters  DVariant=Disabled  IntegratorVariant=Continuous  SatVariant=Enabled  AWVariant=ContClampingIdeal  PCopyVariant=InternalParamsIdeal  TRVariant=Disabled  FdbkBlocksVariant=Forward  IdealPFdbkVariant=Disabled  SatFdbkVariant=Disabled  DerivativeFilterVariant=Disabled  NVariant=Disabled  NCopyVariant=Disabled_SignalSpec  FilterICVariant=Disabled  IntegratorICVariant=InternalICs  ExternalResetVariant=Disabled  TRSumVariant=Passthrough  SumFdbkVariant=Disabled  SumVariant=Sum_PI  TsampFilterVariant=InternalTs  TsampNgainVariant=Passthrough  TsampIntegralVariant=Disabled_SignalSpec  ExternalSaturationOutDataTypeStr=Inherit: Same as second input
  Product : Product
  S_initialize : $bdroot/general/S_initialize  SystemSampleTime=-1  VariantActivationTime=update diagram  AllowFlexibleInterface=on  Latency=0  AutoFrameSizeCalculation=off
  Sum13 : Sum  Inputs=|+-
  Transfer Fcn (with initial states) : Subsystem  mask(Transfer Function with Initial States){N=[1], D=[timeconst 1], X0=0}
      mask prompts: N "Numerator:"; D "Denominator:"; X0 "Initial conditions:"
      mask help: Vector expressions for numerator, and denominator. Coefficients are in descending powers of s.
      mask init:
      | [A,B,C,Dd]=tf2ss(N,D);if (isempty(X0));[m,n]=size(A);X0=zeros(1,m); end;
      mask Help: Specify the initial states for the transfer function.  The state ordering is determined by the m-file tf2ss.  There is no unique mapping of the states in a transfer function to states in a state-space representation.  However, tf2ss will consistently use the same mapping for a given transfer function.
      mask Display: dpoly(N,D,'s')
  convective : Gain  Gain=s_conv  SaturateOnIntegerOverflow=on  OutDataTypeStr=Inherit: Same as input  ParamDataTypeStr=Inherit: Same as input
  maximal power : Constant  Value=max_power
  radiative : Gain  Gain=1-s_conv  SaturateOnIntegerOverflow=on  OutDataTypeStr=Inherit: Same as input  ParamDataTypeStr=Inherit: Same as input
  "[S]" : Outport  VectorParamsAs1DForOutWhenUnconnected=off
  "[HVAC]" : Outport  Port=2  VectorParamsAs1DForOutWhenUnconnected=off
  wires:
  Sum13/1 -> PID/1
  Transfer Fcn (with initial states)/1(Out1) -> Product/1
  convective/1 -> Bus Assignment2/2
  PID/1 -> Transfer Fcn (with initial states)/1(In1)
  maximal power/1 -> Product/2
  temperature room/1 -> Bus Selector5/1
  radiative/1 -> Bus Assignment2/3
  Product/1 -> convective/1, radiative/1, Bus Creator1/1, Integrator/1, Bus Assignment2/4  "heating power"
  Bus Selector5/1 -> Sum13/2  "<Ts>"
  temperature setpoint/1 -> Sum13/1
  Integrator/1 -> Bus Creator1/2  "heating energy"
  Bus Creator1/1 -> "[HVAC]"/1
  S_initialize/1 -> Bus Assignment2/1
  Bus Assignment2/1 -> "[S]"/1

== system carnotUIBK_bus/HVAC/HVAC_1_PHPP/Transfer Fcn (with initial states) ==
  In1 : Inport
  State Space : StateSpace  A=A  B=B  C=C  D=Dd  InitialCondition=X0
  Out1 : Outport  InitialOutput=0  VectorParamsAs1DForOutWhenUnconnected=off
  wires:
  State Space/1 -> Out1/1
  In1/1 -> State Space/1

== system carnotUIBK_bus/HVAC/HVAC_1_PHPP/Transfer Fcn (with initial states)1 ==
  In1 : Inport
  State Space : StateSpace  A=A  B=B  C=C  D=Dd  InitialCondition=X0
  Out1 : Outport  InitialOutput=0  VectorParamsAs1DForOutWhenUnconnected=off
  wires:
  State Space/1 -> Out1/1
  In1/1 -> State Space/1

== system carnotUIBK_bus/HVAC/HVAC_2001_ventilation system simple/ventilation_zone 1 ==
  note: ASSUMPTION: mdot_air_in = mdot_air_out !
  note: AIR VENTILATION outdoors - indoors
  note: x_sup = x_amb + (x_ext - x_amb) * eta_x
  AIB : Inport
  WDB : Inport  Port=2
  Vdot : Inport  Port=3
  Enable : EnablePort
  "\"air\"" : Constant  Value=2
  "1/h -> 1/s" : Gain  Gain=1/3600  SaturateOnIntegerOverflow=on  OutDataTypeStr=Inherit: Same as input  ParamDataTypeStr=Inherit: Same as input
  Bus Assignment2 : BusAssignment  AssignedSignals=Qdotc,mdot_CO2,Qdot_V_mech,mdot_H2O
  Bus Creator1 : BusCreator  Inputs=2
  Bus Selector : BusSelector  OutputSignals=Temperature_Ambient,Relative_Humidity,Station_Pressure
  Bus Selector1 : BusSelector  OutputSignals=Tc,x_H2O,x_CO2
  Constant3 : Constant  Value=1-eta
  Constant5 : Constant  Value=eta_x
  Density : carnot/Basic/Material_Properties/Density  VariantControl=CarlibClassic  INPUTARGUMENTS=state variables (classic)  DEBUGLEVEL=NOLEVEL  MAXTOTALWARNINGS=inf  MAXCONSECUTIVEWARNINGS=inf  WRITETOFILE=0  FILENAME='errors.txt'
      settings: SourceProductName=Carnot
  Fcn : Fcn  Expr=u / (1+u)
  Fcn1 : Fcn  Expr=u / (1+u)
  Integrator : Integrator
  Mux1 : Mux  Inputs=[1 1]
  Mux4 : Mux  Inputs=2
  Product1 : Product  InputSameDT=on  SaturateOnIntegerOverflow=on  OutDataTypeStr=Inherit: Same as first input
  Product2 : Product  InputSameDT=on  SaturateOnIntegerOverflow=on  OutDataTypeStr=Inherit: Same as first input
  Product3 : Product  InputSameDT=on  SaturateOnIntegerOverflow=on  OutDataTypeStr=Inherit: Same as first input
  Product4 : Product  Inputs=4  InputSameDT=on  SaturateOnIntegerOverflow=on  OutDataTypeStr=Inherit: Same as first input
  RelHum2x : carnot/Basic/Material_Properties/RelHum2x
      settings: SourceProductName=Carnot
  S_initialize : $bdroot/general/S_initialize  SystemSampleTime=-1  VariantActivationTime=update diagram  AllowFlexibleInterface=on  Latency=0  AutoFrameSizeCalculation=off
  Subsystem : Subsystem
  Sum : Sum  Inputs=-+  InputSameDT=on  SaturateOnIntegerOverflow=on  OutDataTypeStr=Inherit: Same as first input
  Sum1 : Sum  Inputs=-+  InputSameDT=on  SaturateOnIntegerOverflow=on  OutDataTypeStr=Inherit: Same as first input
  Sum2 : Sum  Inputs=++-  InputSameDT=on  SaturateOnIntegerOverflow=on  OutDataTypeStr=Inherit: Same as first input
  Terminator : Terminator
  cp Constant : Constant  Value=1006.8
  rho(CO2) / rho(air) * CO2norm (kg/kg) : Constant  Value=1.529*CO2norm
  "[S]" : Outport  VectorParamsAs1DForOutWhenUnconnected=off
  "[HVAC]" : Outport  Port=2  VectorParamsAs1DForOutWhenUnconnected=off
  wires:
  Fcn1/1 -> Sum2/1, Sum1/1
  Fcn/1 -> Sum1/2, Sum2/3
  Product2/1 -> Bus Assignment2/5  "mdot_H2O"
  Sum2/1 -> Product2/2  "x_sup"
  Product1/1 -> Sum2/2
  Sum1/1 -> Product1/2
  Constant5/1 -> Product1/1
  Subsystem/1(mdot_H2O) -> Terminator/1  "mdot_H2O"
  Vdot/1 -> "1/h -> 1/s"/1
  Subsystem/2(mdot_CO2) -> Bus Assignment2/3  "mdot_CO2"
  WDB/1 -> Bus Selector/1
  AIB/1 -> Bus Selector1/1
  Density/1 -> Product3/2
  Bus Selector/3 -> RelHum2x/2, Density/2  "<Station_Pressure>"
  Bus Selector/2 -> RelHum2x/3  "<Relative_Humidity>"
  Bus Selector/1 -> RelHum2x/1, Density/1, Sum/2  "<Temperature_Ambient>"
  RelHum2x/1 -> Density/4, Mux4/1, Fcn1/1  "x_H2O"
  "\"air\""/1 -> Density/3
  Mux1/1 -> Subsystem/2(x_in)  "[x_H2O, x_CO2]_in"
  Bus Selector1/1 -> Sum/1  "<Tc>"
  Mux4/1 -> Subsystem/3(x_out)
  rho(CO2) / rho(air) * CO2norm (kg/kg)/1 -> Mux4/2  "x_CO2"
  Sum/1 -> Product4/2  "dT"
  cp Constant/1 -> Product4/3  "cp"
  Product3/1 -> Product4/4, Product2/1, Subsystem/1(mdot_air)
  Bus Selector1/2 -> Mux1/1, Fcn/1  "<x_H2O>"
  Bus Selector1/3 -> Mux1/2  "<x_CO2>"
  Constant3/1 -> Product4/1
  "1/h -> 1/s"/1 -> Product3/1
  Bus Creator1/1 -> "[HVAC]"/1
  Product4/1 -> Bus Assignment2/2, Bus Assignment2/4, Integrator/1, Bus Creator1/1  "ventilation power"
  Integrator/1 -> Bus Creator1/2  "ventilation energy"
  S_initialize/1 -> Bus Assignment2/1
  Bus Assignment2/1 -> "[S]"/1

== system carnotUIBK_bus/HVAC/HVAC_9001_window shading/Transfer Fcn (with initial states) ==
  In1 : Inport
  State Space : StateSpace  A=A  B=B  C=C  D=Dd  InitialCondition=X0
  Out1 : Outport  InitialOutput=0  VectorParamsAs1DForOutWhenUnconnected=off
  wires:
  In1/1 -> State Space/1
  State Space/1 -> Out1/1

== system carnotUIBK_bus/HVAC/HVAC_9002_window opening/window opening 1 ==
  setpoint : Inport
  AIB : Inport  Port=2
  WDB : Inport  Port=3
  Enable : EnablePort
  Add : Sum
  Bus Selector1 : BusSelector  OutputSignals=Temperature_Ambient
  Bus Selector5 : BusSelector  OutputSignals=Ts,Tc,p,x_H2O
  Product : Product
  Saturation : Saturate  UpperLimit=1  LowerLimit=0
  Sum : Sum  Inputs=|-+
  Sum1 : Sum  Inputs=|+-
  Sum2 : Sum  Inputs=|-+
  Transfer Fcn (with initial states) : Subsystem  mask(Transfer Function with Initial States){N=[1], D=[600 1], X0=0}
      mask prompts: N "Numerator:"; D "Denominator:"; X0 "Initial conditions:"
      mask help: Vector expressions for numerator, and denominator. Coefficients are in descending powers of s.
      mask init:
      | [A,B,C,Dd]=tf2ss(N,D);if (isempty(X0));[m,n]=size(A);X0=zeros(1,m); end;
      mask Help: Specify the initial states for the transfer function.  The state ordering is determined by the m-file tf2ss.  There is no unique mapping of the states in a transfer function to states in a state-space representation.  However, tf2ss will consistently use the same mapping for a given transfer function.
      mask Display: dpoly(N,D,'s')
  Transfer Fcn (with initial states)1 : Subsystem  mask(Transfer Function with Initial States){N=[1], D=[600 1], X0=0}
      mask prompts: N "Numerator:"; D "Denominator:"; X0 "Initial conditions:"
      mask help: Vector expressions for numerator, and denominator. Coefficients are in descending powers of s.
      mask init:
      | [A,B,C,Dd]=tf2ss(N,D);if (isempty(X0));[m,n]=size(A);X0=zeros(1,m); end;
      mask Help: Specify the initial states for the transfer function.  The state ordering is determined by the m-file tf2ss.  There is no unique mapping of the states in a transfer function to states in a state-space representation.  However, tf2ss will consistently use the same mapping for a given transfer function.
      mask Display: dpoly(N,D,'s')
  Transfer Fcn (with initial states)2 : Subsystem  mask(Transfer Function with Initial States){N=[1], D=[600 1], X0=0}
      mask prompts: N "Numerator:"; D "Denominator:"; X0 "Initial conditions:"
      mask help: Vector expressions for numerator, and denominator. Coefficients are in descending powers of s.
      mask init:
      | [A,B,C,Dd]=tf2ss(N,D);if (isempty(X0));[m,n]=size(A);X0=zeros(1,m); end;
      mask Help: Specify the initial states for the transfer function.  The state ordering is determined by the m-file tf2ss.  There is no unique mapping of the states in a transfer function to states in a state-space representation.  However, tf2ss will consistently use the same mapping for a given transfer function.
      mask Display: dpoly(N,D,'s')
  on/off ambient : Relay  OnSwitchValue=0.5  OffSwitchValue=-0.5
  on/off hum : Relay  OnSwitchValue=0.5  OffSwitchValue=-0.5
  on/off roomtemp : Relay  OnSwitchValue=0.5  OffSwitchValue=-0.5
  setpoint humidity : Constant  Value=85
  x2RelHum_UIBK : carnot/Basic/Material_Properties/x2RelHum
      settings: SourceProductName=Carnot
  state : Outport  VectorParamsAs1DForOutWhenUnconnected=off
  wires:
  AIB/1 -> Bus Selector5/1
  setpoint/1 -> Sum/1
  Bus Selector5/1 -> Transfer Fcn (with initial states)/1(In1)  "<Ts>"
  Sum/1 -> on/off roomtemp/1
  on/off roomtemp/1 -> Product/1
  WDB/1 -> Bus Selector1/1
  Bus Selector1/1 -> Transfer Fcn (with initial states)2/1(In1)  "<Temperature_Ambient>"
  Sum1/1 -> on/off ambient/1
  on/off ambient/1 -> Product/2
  Bus Selector5/2 -> x2RelHum_UIBK/1  "<Tc>"
  Bus Selector5/3 -> x2RelHum_UIBK/2  "<p>"
  Bus Selector5/4 -> x2RelHum_UIBK/3  "<x_H2O>"
  Sum2/1 -> on/off hum/1
  x2RelHum_UIBK/1 -> Transfer Fcn (with initial states)1/1(In1)
  setpoint humidity/1 -> Sum2/1
  Add/1 -> Saturation/1
  Product/1 -> Add/2
  on/off hum/1 -> Add/1
  Saturation/1 -> state/1
  Transfer Fcn (with initial states)/1(Out1) -> Sum1/1, Sum/2
  Transfer Fcn (with initial states)2/1(Out1) -> Sum1/2
  Transfer Fcn (with initial states)1/1(Out1) -> Sum2/2
